simulink model "REPLAY_TRADITIONAL_21"  (R2021a)
settings: Solver=ode23tb  StartTime=0.0  StopTime=27  MaxStep=1/60  RelTol=1e-2  AbsTol=1e-1  EnableMultiTasking=on
PreLoadFcn:
  | NE39bus_data;
  | PSSMODEL=1;
  | LPSS=0;
  | WAPSS=0;
  | WAPSS2=0;
undefined symbols (not defined in the file): AVR_Data, D1, Delta, line, mac_con, MB, Ns, p0, Pn, s
libraries: spsThreePhaseVIMeasurementLib x40, spsThreePhasePISectionLineLib x34, spsGenericPowerSystemStabilizerLib x20, spsThreePhaseParallelRLCLoadLib x14, spsThreePhaseTransformerTwoWindingsLib x12, spsSynchronousMachinepuStandardLib x10, spsExcitationSystemLib x10, spsMultiBandPowerSystemStabilizerLib x10, spsSteamTurbineandGovernorLib x10, slpidlib x10, spsLoadFlowBusLib x9, spsThreePhaseBreakerLib x8
(part 2 of 4)

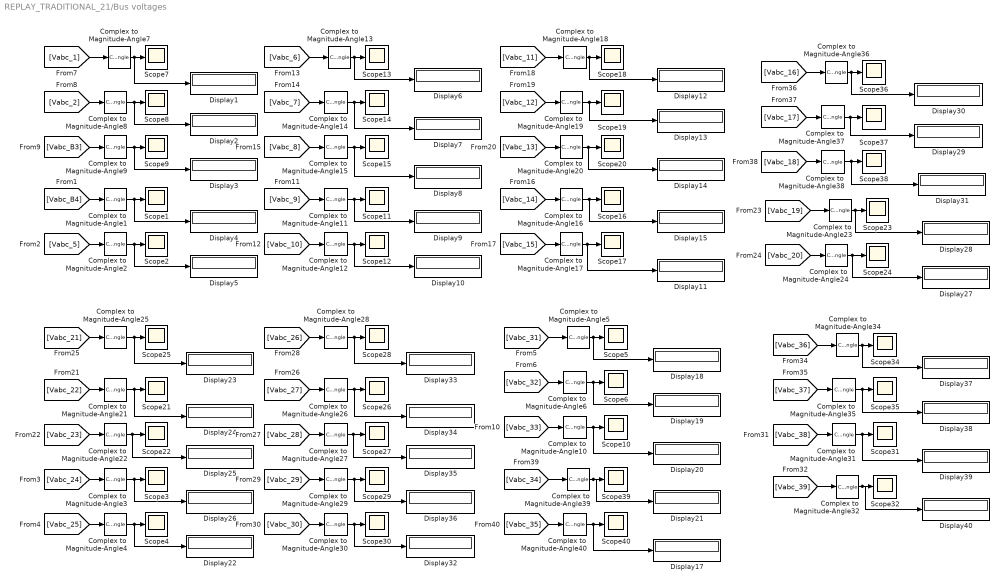
== system REPLAY_TRADITIONAL_21/Bus voltages ==
  Complex to Magnitude-Angle{1..32,34..40} (39 alike) : ComplexToMagnitudeAngle  Output=Magnitude
  Display{1..15,17..40} (39 alike) : Display
  Scope{1..32,34..40} (39 alike) : Scope
  wires:
  [Vabc_1] -> Complex to Magnitude-Angle7/1
  Complex to Magnitude-Angle7/1 -> Display1/1, Scope7/1
  [Vabc_2] -> Complex to Magnitude-Angle8/1
  Complex to Magnitude-Angle8/1 -> Display2/1, Scope8/1
  [Vabc_B3] -> Complex to Magnitude-Angle9/1
  Complex to Magnitude-Angle9/1 -> Display3/1, Scope9/1
  [Vabc_B4] -> Complex to Magnitude-Angle1/1
  Complex to Magnitude-Angle1/1 -> Display4/1, Scope1/1
  [Vabc_5] -> Complex to Magnitude-Angle2/1
  Complex to Magnitude-Angle2/1 -> Display5/1, Scope2/1
  [Vabc_31] -> Complex to Magnitude-Angle5/1
  [Vabc_32] -> Complex to Magnitude-Angle6/1
  [Vabc_33] -> Complex to Magnitude-Angle10/1
  [Vabc_24] -> Complex to Magnitude-Angle3/1
  [Vabc_25] -> Complex to Magnitude-Angle4/1
  [Vabc_6] -> Complex to Magnitude-Angle13/1
  [Vabc_7] -> Complex to Magnitude-Angle14/1
  [Vabc_8] -> Complex to Magnitude-Angle15/1
  [Vabc_9] -> Complex to Magnitude-Angle11/1
  [Vabc_10] -> Complex to Magnitude-Angle12/1
  [Vabc_11] -> Complex to Magnitude-Angle18/1
  Complex to Magnitude-Angle18/1 -> Display12/1, Scope18/1
  [Vabc_12] -> Complex to Magnitude-Angle19/1
  [Vabc_13] -> Complex to Magnitude-Angle20/1
  Complex to Magnitude-Angle20/1 -> Display14/1, Scope20/1
  [Vabc_14] -> Complex to Magnitude-Angle16/1
  Complex to Magnitude-Angle16/1 -> Display15/1, Scope16/1
  [Vabc_15] -> Complex to Magnitude-Angle17/1
  Complex to Magnitude-Angle17/1 -> Display11/1, Scope17/1
  [Vabc_19] -> Complex to Magnitude-Angle23/1
  [Vabc_20] -> Complex to Magnitude-Angle24/1
  [Vabc_21] -> Complex to Magnitude-Angle25/1
  [Vabc_22] -> Complex to Magnitude-Angle21/1
  [Vabc_23] -> Complex to Magnitude-Angle22/1
  Complex to Magnitude-Angle13/1 -> Display6/1, Scope13/1
  Complex to Magnitude-Angle14/1 -> Display7/1, Scope14/1
  Complex to Magnitude-Angle15/1 -> Display8/1, Scope15/1
  Complex to Magnitude-Angle11/1 -> Display9/1, Scope11/1
  Complex to Magnitude-Angle12/1 -> Display10/1, Scope12/1
  Complex to Magnitude-Angle19/1 -> Display13/1, Scope19/1
  [Vabc_16] -> Complex to Magnitude-Angle36/1
  [Vabc_17] -> Complex to Magnitude-Angle37/1
  [Vabc_18] -> Complex to Magnitude-Angle38/1
  Complex to Magnitude-Angle38/1 -> Display31/1, Scope38/1
  [Vabc_34] -> Complex to Magnitude-Angle39/1
  [Vabc_35] -> Complex to Magnitude-Angle40/1
  Complex to Magnitude-Angle5/1 -> Display18/1, Scope5/1
  Complex to Magnitude-Angle10/1 -> Display20/1, Scope10/1
  Complex to Magnitude-Angle39/1 -> Display21/1, Scope39/1
  Complex to Magnitude-Angle40/1 -> Display17/1, Scope40/1
  Complex to Magnitude-Angle6/1 -> Display19/1, Scope6/1
  Complex to Magnitude-Angle25/1 -> Display23/1, Scope25/1
  Complex to Magnitude-Angle22/1 -> Display25/1, Scope22/1
  Complex to Magnitude-Angle3/1 -> Display26/1, Scope3/1
  Complex to Magnitude-Angle4/1 -> Display22/1, Scope4/1
  Complex to Magnitude-Angle21/1 -> Display24/1, Scope21/1
  Complex to Magnitude-Angle23/1 -> Display28/1, Scope23/1
  Complex to Magnitude-Angle24/1 -> Display27/1, Scope24/1
  Complex to Magnitude-Angle36/1 -> Display30/1, Scope36/1
  Complex to Magnitude-Angle37/1 -> Display29/1, Scope37/1
  [Vabc_29] -> Complex to Magnitude-Angle29/1
  [Vabc_30] -> Complex to Magnitude-Angle30/1
  [Vabc_26] -> Complex to Magnitude-Angle28/1
  [Vabc_27] -> Complex to Magnitude-Angle26/1
  [Vabc_28] -> Complex to Magnitude-Angle27/1
  Complex to Magnitude-Angle28/1 -> Display33/1, Scope28/1
  Complex to Magnitude-Angle27/1 -> Display35/1, Scope27/1
  Complex to Magnitude-Angle29/1 -> Display36/1, Scope29/1
  Complex to Magnitude-Angle30/1 -> Display32/1, Scope30/1
  Complex to Magnitude-Angle26/1 -> Display34/1, Scope26/1
  [Vabc_36] -> Complex to Magnitude-Angle34/1
  [Vabc_37] -> Complex to Magnitude-Angle35/1
  [Vabc_38] -> Complex to Magnitude-Angle31/1
  [Vabc_39] -> Complex to Magnitude-Angle32/1
  Complex to Magnitude-Angle34/1 -> Display37/1, Scope34/1
  Complex to Magnitude-Angle31/1 -> Display39/1, Scope31/1
  Complex to Magnitude-Angle32/1 -> Display40/1, Scope32/1
  Complex to Magnitude-Angle35/1 -> Display38/1, Scope35/1

== system REPLAY_TRADITIONAL_21/G1 ==
  DFG1 : Inport
  Bus Selector : BusSelector  OutputSignals="Mechanical.Rotor speed deviation  dw (pu)"
  Bus to Vector : BusToVector
  Fcn2 : Fcn  Expr=60*(1+u)
  G1 : spsSynchronousMachinepuStandardLib/Synchronous Machine pu Standard  PresetModel=No  MechanicalLoad=Mechanical power Pm  ShowDetailedParameters=on  RotorType=Round  Units=per unit standard parameters  MeasurementBus=off  NominalParameters="[Pn(1,1)*1E9  345000   50 ]"  Reactances1="[mac_con(1,6:8)  mac_con(1,11:13)  mac_con(1,4)]"  Reactances2=[ 1.305, 0.296, 0.252, 0.474, 0.243, 0.18 ]  dAxisTimeConstants=Open-circuit  qAxisTimeConstants=Open-circuit  TimeConstants1=[]  TimeConstants2="[mac_con(1,9:10)  mac_con(1,14:15)]"  TimeConstants3=[]  TimeConstants4=[]  TimeConstants5=[ 1.01, 0.053, 0.1 ]  TimeConstants6=[]  TimeConstants7=[]  TimeConstants8=[]  StatorResistance=mac_con(1,5)  Mechanical="[ mac_con(1,16)  0  4]"  PolePairs=4  InitialConditions=[0 -53.3817 1.03438 1.03438 1.03438 11.5505 -108.45 131.55 1.07168]  SetSaturation=off  Saturation=[0.6404,0.7127,0.8441,0.9214,0.9956,1.082,1.19,1.316,1.457;0.7,0.7698,0.8872,0.9466,0.9969,1.046,1.1,1.151,1.201]  LoadFlowParameters=[1 1000000000 0 0 0]  TsPowergui=0  TsBlock=-1  IterativeModel=Forward Euler  IterativeDiscreteModel=Trapezoidal non iterative  BusType=PV  Pref=p0(1,1)*1E9  Qref=0  Qmin=-inf  Qmax=inf  PLF=0  QLF=0
      settings: SourceProductBaseCode=PS
  M1: Turbine & Regulators : Subsystem
  Matrix Multiply1 : Product  Multiplication=Matrix(*)
  Matrix Multiply2 : Product  Multiplication=Matrix(*)
  PID Controller : slpidlib/PID Controller  Controller=PID  Form=Parallel  TimeDomain=Continuous-time  UseExternalTs=off  SampleTime=-1  IntegratorMethod=Forward Euler  FilterMethod=Forward Euler  ControllerParametersSource=internal  P=-0.20298  I=1  D=0  UseFilter=on  N=100  TunerSelectOption=Frequency Response Based  InitialConditionSource=internal  InitialConditionForIntegrator=0  InitialConditionForFilter=0  DifferentiatorICPrevScaledInput=0  ExternalReset=none  TrackingMode=off  Kt=1  LimitOutput=off  SatLimitsSource=internal  UpperSaturationLimit=inf  LowerSaturationLimit=-inf  LinearizeAsGain=on  AntiWindupMode=none  Kb=1  POutMin=[]  POutMax=[]  IOutMin=[]  IOutMax=[]  DOutMin=[]  DOutMax=[]  NOutMin=[]  NOutMax=[]  SumOutMin=[]  SumOutMax=[]  SaturationOutMin=[]  SaturationOutMax=[]  PParamMin=[]  PParamMax=[]  IParamMin=[]  IParamMax=[]  DParamMin=[]  DParamMax=[]  NParamMin=[]  NParamMax=[]  KbParamMin=[]  KbParamMax=[]  KtParamMin=[]  KtParamMax=[]  KbOutMin=[]  KbOutMax=[]  KtOutMin=[]  KtOutMax=[]  IntegratorOutMin=[]  IntegratorOutMax=[]  FilterOutMin=[]  FilterOutMax=[]  SumI1OutMin=[]  SumI1OutMax=[]  SumI2OutMin=[]  SumI2OutMax=[]  SumI3OutMin=[]  SumI3OutMax=[]  SumI4OutMin=[]  SumI4OutMax=[]  SumDOutMin=[]  SumDOutMax=[]  DifferentiatorOutMin=[]  DifferentiatorOutMax=[]  FilterDiffOutCoefMin=[]  FilterDiffOutCoefMax=[]  ReciprocalOutMin=[]  ReciprocalOutMax=[]  SumDenOutMin=[]  SumDenOutMax=[]  SumNumOutMin=[]  SumNumOutMax=[]  DivideOutMin=[]  DivideOutMax=[]  UdiffTsProdOutMin=[]  UdiffTsProdOutMax=[]  NTsProdOutMin=[]  NTsProdOutMax=[]  UintegralTsProdOutMin=[]  UintegralTsProdOutMax=[]  UngainTsProdOutMin=[]  UngainTsProdOutMax=[]  IntegratorContinuousStateAttributes=''  IntegratorStateMustResolveToSignalObject=off  IntegratorRTWStateStorageClass=Auto  FilterContinuousStateAttributes=''  FilterStateMustResolveToSignalObject=off  FilterRTWStateStorageClass=Auto  ParallelPVariant=InternalParameters  IdealPVariant=Disabled  IVariant=InternalParameters  DVariant=InternalParameters  IntegratorVariant=Continuous  SatVariant=Disabled  AWVariant=Passthrough  PCopyVariant=Disabled  TRVariant=Disabled  FdbkBlocksVariant=Forward  IdealPFdbkVariant=Disabled  SatFdbkVariant=Disabled  DerivativeFilterVariant=ContFilter  NVariant=InternalParameters  NCopyVariant=Disabled  FilterICVariant=InternalICsFilter  IntegratorICVariant=InternalICs  ExternalResetVariant=Disabled  TRSumVariant=Passthrough  SumFdbkVariant=Disabled  SumVariant=Sum_PID  TsampFilterVariant=InternalTs  TsampNgainVariant=Passthrough  TsampIntegralVariant=Passthrough  ExternalSaturationOutDataTypeStr=Inherit: Same as second input
  Pref1 : Constant
  Scope3 : Scope
  Sum : Sum  Inputs=|++
  To Workspace : ToWorkspace  VariableName=average_frequency_39_bus  SaveFormat=Timeseries  SampleTime=-1
  Vref1 : Constant
  A : PMIOPort  Side=Left
  B : PMIOPort  Port=2  Side=Left
  C : PMIOPort  Port=3  Side=Left
  GEN1 : Outport
  wires:
  [PSSmodel] -> M1: Turbine & Regulators/4(PSS1)
  PID Controller/1 -> Sum/2
  Sum/1 -> M1: Turbine & Regulators/2(Pref1)
  Pref1/1 -> Sum/1
  Vref1/1 -> M1: Turbine & Regulators/3(Vref1)
  G1/1 -> Bus to Vector/1, M1: Turbine & Regulators/1(m), Bus Selector/1
  Bus Selector/1 -> Fcn2/1, PID Controller/1  "<Rotor speed deviation  dw (pu)>"
  Fcn2/1 -> GEN1/1, Scope3/1, To Workspace/1
  DFG1/1 -> Matrix Multiply1/1, Matrix Multiply2/1
  M1: Turbine & Regulators/1(Pm1) -> Matrix Multiply1/2
  Matrix Multiply1/1 -> G1/1
  M1: Turbine & Regulators/2(Vf1) -> Matrix Multiply2/2
  Matrix Multiply2/1 -> G1/2
  connections:
  A/RConn1 -- G1/RConn1
  B/RConn1 -- G1/RConn2
  C/RConn1 -- G1/RConn3

== system REPLAY_TRADITIONAL_21/G10 ==
  Inport : Inport
  Bus Selector : BusSelector  OutputSignals="Mechanical.Rotor speed deviation  dw (pu)"
  Fcn2 : Fcn  Expr=60*(1+u)
  G10 : spsSynchronousMachinepuStandardLib/Synchronous Machine pu Standard  PresetModel=No  MechanicalLoad=Mechanical power Pm  ShowDetailedParameters=on  RotorType=Round  Units=per unit standard parameters  MeasurementBus=off  NominalParameters="[Pn(10,1)*1E9  22000   50 ]"  Reactances1="[mac_con(10,6:8)  mac_con(10,11:13)  mac_con(10,4)]"  Reactances2=[ 1.305, 0.296, 0.252, 0.474, 0.243, 0.18 ]  dAxisTimeConstants=Open-circuit  qAxisTimeConstants=Open-circuit  TimeConstants1=[]  TimeConstants2="[mac_con(10,9:10)  mac_con(10,14:15)]"  TimeConstants3=[]  TimeConstants4=[]  TimeConstants5=[ 1.01, 0.053, 0.1 ]  TimeConstants6=[]  TimeConstants7=[]  TimeConstants8=[]  StatorResistance=mac_con(10,5)  Mechanical="[ mac_con(10,16)  0  4]"  PolePairs=4  InitialConditions=[0 -76.9944 0.265611 0.265611 0.265611 -15.9627 -135.963 104.037 1.1157]  SetSaturation=off  Saturation=[0.6404,0.7127,0.8441,0.9214,0.9956,1.082,1.19,1.316,1.457;0.7,0.7698,0.8872,0.9466,0.9969,1.046,1.1,1.151,1.201]  LoadFlowParameters=[1 250000000 0 0 0]  TsPowergui=0  TsBlock=-1  IterativeModel=Forward Euler  IterativeDiscreteModel=Trapezoidal non iterative  BusType=PV  Pref=p0(10,1)*1E9  Qref=0  Qmin=-inf  Qmax=inf  PLF=0  QLF=0
      settings: SourceProductBaseCode=PS
  M10: Turbine & Regulators : Subsystem
  Matrix Multiply1 : Product  Multiplication=Matrix(*)
  Matrix Multiply2 : Product  Multiplication=Matrix(*)
  PID Controller : slpidlib/PID Controller  Controller=PID  Form=Parallel  TimeDomain=Continuous-time  UseExternalTs=off  SampleTime=-1  IntegratorMethod=Forward Euler  FilterMethod=Forward Euler  ControllerParametersSource=internal  P=-0.20298  I=1  D=0  UseFilter=on  N=100  TunerSelectOption=Frequency Response Based  InitialConditionSource=internal  InitialConditionForIntegrator=0  InitialConditionForFilter=0  DifferentiatorICPrevScaledInput=0  ExternalReset=none  TrackingMode=off  Kt=1  LimitOutput=off  SatLimitsSource=internal  UpperSaturationLimit=inf  LowerSaturationLimit=-inf  LinearizeAsGain=on  AntiWindupMode=none  Kb=1  POutMin=[]  POutMax=[]  IOutMin=[]  IOutMax=[]  DOutMin=[]  DOutMax=[]  NOutMin=[]  NOutMax=[]  SumOutMin=[]  SumOutMax=[]  SaturationOutMin=[]  SaturationOutMax=[]  PParamMin=[]  PParamMax=[]  IParamMin=[]  IParamMax=[]  DParamMin=[]  DParamMax=[]  NParamMin=[]  NParamMax=[]  KbParamMin=[]  KbParamMax=[]  KtParamMin=[]  KtParamMax=[]  KbOutMin=[]  KbOutMax=[]  KtOutMin=[]  KtOutMax=[]  IntegratorOutMin=[]  IntegratorOutMax=[]  FilterOutMin=[]  FilterOutMax=[]  SumI1OutMin=[]  SumI1OutMax=[]  SumI2OutMin=[]  SumI2OutMax=[]  SumI3OutMin=[]  SumI3OutMax=[]  SumI4OutMin=[]  SumI4OutMax=[]  SumDOutMin=[]  SumDOutMax=[]  DifferentiatorOutMin=[]  DifferentiatorOutMax=[]  FilterDiffOutCoefMin=[]  FilterDiffOutCoefMax=[]  ReciprocalOutMin=[]  ReciprocalOutMax=[]  SumDenOutMin=[]  SumDenOutMax=[]  SumNumOutMin=[]  SumNumOutMax=[]  DivideOutMin=[]  DivideOutMax=[]  UdiffTsProdOutMin=[]  UdiffTsProdOutMax=[]  NTsProdOutMin=[]  NTsProdOutMax=[]  UintegralTsProdOutMin=[]  UintegralTsProdOutMax=[]  UngainTsProdOutMin=[]  UngainTsProdOutMax=[]  IntegratorContinuousStateAttributes=''  IntegratorStateMustResolveToSignalObject=off  IntegratorRTWStateStorageClass=Auto  FilterContinuousStateAttributes=''  FilterStateMustResolveToSignalObject=off  FilterRTWStateStorageClass=Auto  ParallelPVariant=InternalParameters  IdealPVariant=Disabled  IVariant=InternalParameters  DVariant=InternalParameters  IntegratorVariant=Continuous  SatVariant=Disabled  AWVariant=Passthrough  PCopyVariant=Disabled  TRVariant=Disabled  FdbkBlocksVariant=Forward  IdealPFdbkVariant=Disabled  SatFdbkVariant=Disabled  DerivativeFilterVariant=ContFilter  NVariant=InternalParameters  NCopyVariant=Disabled  FilterICVariant=InternalICsFilter  IntegratorICVariant=InternalICs  ExternalResetVariant=Disabled  TRSumVariant=Passthrough  SumFdbkVariant=Disabled  SumVariant=Sum_PID  TsampFilterVariant=InternalTs  TsampNgainVariant=Passthrough  TsampIntegralVariant=Passthrough  ExternalSaturationOutDataTypeStr=Inherit: Same as second input
  Pref10 : Constant  Value=0.25
  Scope : Scope
  Sum : Sum  Inputs=|+-
  Vref10 : Constant
  A : PMIOPort  Side=Left
  B : PMIOPort  Port=2  Side=Left
  C : PMIOPort  Port=3  Side=Left
  "GEN10 " : Outport
  wires:
  [PSSmodel] -> M10: Turbine & Regulators/4(PSS10)
  Vref10/1 -> M10: Turbine & Regulators/3(Vref10)
  G10/1 -> Bus Selector/1, M10: Turbine & Regulators/1(m)
  Bus Selector/1 -> PID Controller/1, Fcn2/1  "<Rotor speed deviation  dw (pu)>"
  Sum/1 -> M10: Turbine & Regulators/2(Pref10)
  Pref10/1 -> Sum/1
  PID Controller/1 -> Sum/2
  Fcn2/1 -> "GEN10 "/1, Scope/1
  Inport/1 -> Matrix Multiply2/1, Matrix Multiply1/1
  M10: Turbine & Regulators/1(Pm10) -> Matrix Multiply1/2
  Matrix Multiply1/1 -> G10/1
  M10: Turbine & Regulators/2(Vf10) -> Matrix Multiply2/2
  Matrix Multiply2/1 -> G10/2
  connections:
  A/RConn1 -- G10/RConn1
  B/RConn1 -- G10/RConn2
  C/RConn1 -- G10/RConn3

== system REPLAY_TRADITIONAL_21/G2 ==
  DFG2 : Inport
  Bus Selector : BusSelector  OutputSignals="Mechanical.Rotor speed deviation  dw (pu)"
  Fcn2 : Fcn  Expr=60*(1+u)
  G2 : spsSynchronousMachinepuStandardLib/Synchronous Machine pu Standard  PresetModel=No  MechanicalLoad=Mechanical power Pm  ShowDetailedParameters=on  RotorType=Round  Units=per unit standard parameters  MeasurementBus=off  NominalParameters="[Pn(2,1)*1E9  22000   50 ]"  Reactances1="[mac_con(2,6:8)  mac_con(2,11:13)  mac_con(2,4)]"  Reactances2=[ 1.305, 0.296, 0.252, 0.474, 0.243, 0.18 ]  dAxisTimeConstants=Open-circuit  qAxisTimeConstants=Open-circuit  TimeConstants1=[]  TimeConstants2="[mac_con(2,9:10)  mac_con(2,14:15)]"  TimeConstants3=[]  TimeConstants4=[]  TimeConstants5=[ 1.01, 0.053, 0.1 ]  TimeConstants6=[]  TimeConstants7=[]  TimeConstants8=[]  StatorResistance=mac_con(2,5)  Mechanical="[ mac_con(2,16)  0  4]"  PolePairs=4  InitialConditions=[0 -63.2657 0.339533 0.339533 0.339533 -35.2425 -155.242 84.7575 1.77729]  SetSaturation=off  Saturation=[0.6404,0.7127,0.8441,0.9214,0.9956,1.082,1.19,1.316,1.457;0.7,0.7698,0.8872,0.9466,0.9969,1.046,1.1,1.151,1.201]  LoadFlowParameters=[2 546000000 0 0 0]  TsPowergui=0  TsBlock=-1  IterativeModel=Forward Euler  IterativeDiscreteModel=Trapezoidal non iterative  BusType=swing  Pref=0  Qref=0  Qmin=-inf  Qmax=inf  PLF=0  QLF=0
      settings: SourceProductBaseCode=PS
  M2: Turbine & Regulators : Subsystem
  Matrix Multiply1 : Product  Multiplication=Matrix(*)
  Matrix Multiply2 : Product  Multiplication=Matrix(*)
  PID Controller : slpidlib/PID Controller  Controller=PID  Form=Parallel  TimeDomain=Continuous-time  UseExternalTs=off  SampleTime=-1  IntegratorMethod=Forward Euler  FilterMethod=Forward Euler  ControllerParametersSource=internal  P=-0.20298  I=1  D=0  UseFilter=on  N=100  TunerSelectOption=Frequency Response Based  InitialConditionSource=internal  InitialConditionForIntegrator=0  InitialConditionForFilter=0  DifferentiatorICPrevScaledInput=0  ExternalReset=none  TrackingMode=off  Kt=1  LimitOutput=off  SatLimitsSource=internal  UpperSaturationLimit=inf  LowerSaturationLimit=-inf  LinearizeAsGain=on  AntiWindupMode=none  Kb=1  POutMin=[]  POutMax=[]  IOutMin=[]  IOutMax=[]  DOutMin=[]  DOutMax=[]  NOutMin=[]  NOutMax=[]  SumOutMin=[]  SumOutMax=[]  SaturationOutMin=[]  SaturationOutMax=[]  PParamMin=[]  PParamMax=[]  IParamMin=[]  IParamMax=[]  DParamMin=[]  DParamMax=[]  NParamMin=[]  NParamMax=[]  KbParamMin=[]  KbParamMax=[]  KtParamMin=[]  KtParamMax=[]  KbOutMin=[]  KbOutMax=[]  KtOutMin=[]  KtOutMax=[]  IntegratorOutMin=[]  IntegratorOutMax=[]  FilterOutMin=[]  FilterOutMax=[]  SumI1OutMin=[]  SumI1OutMax=[]  SumI2OutMin=[]  SumI2OutMax=[]  SumI3OutMin=[]  SumI3OutMax=[]  SumI4OutMin=[]  SumI4OutMax=[]  SumDOutMin=[]  SumDOutMax=[]  DifferentiatorOutMin=[]  DifferentiatorOutMax=[]  FilterDiffOutCoefMin=[]  FilterDiffOutCoefMax=[]  ReciprocalOutMin=[]  ReciprocalOutMax=[]  SumDenOutMin=[]  SumDenOutMax=[]  SumNumOutMin=[]  SumNumOutMax=[]  DivideOutMin=[]  DivideOutMax=[]  UdiffTsProdOutMin=[]  UdiffTsProdOutMax=[]  NTsProdOutMin=[]  NTsProdOutMax=[]  UintegralTsProdOutMin=[]  UintegralTsProdOutMax=[]  UngainTsProdOutMin=[]  UngainTsProdOutMax=[]  IntegratorContinuousStateAttributes=''  IntegratorStateMustResolveToSignalObject=off  IntegratorRTWStateStorageClass=Auto  FilterContinuousStateAttributes=''  FilterStateMustResolveToSignalObject=off  FilterRTWStateStorageClass=Auto  ParallelPVariant=InternalParameters  IdealPVariant=Disabled  IVariant=InternalParameters  DVariant=InternalParameters  IntegratorVariant=Continuous  SatVariant=Disabled  AWVariant=Passthrough  PCopyVariant=Disabled  TRVariant=Disabled  FdbkBlocksVariant=Forward  IdealPFdbkVariant=Disabled  SatFdbkVariant=Disabled  DerivativeFilterVariant=ContFilter  NVariant=InternalParameters  NCopyVariant=Disabled  FilterICVariant=InternalICsFilter  IntegratorICVariant=InternalICs  ExternalResetVariant=Disabled  TRSumVariant=Passthrough  SumFdbkVariant=Disabled  SumVariant=Sum_PID  TsampFilterVariant=InternalTs  TsampNgainVariant=Passthrough  TsampIntegralVariant=Passthrough  ExternalSaturationOutDataTypeStr=Inherit: Same as second input
  Pref2 : Constant  Value=0.277303
  Scope : Scope
  Sum : Sum  Inputs=|+-
  Vref2 : Constant
  A : PMIOPort  Side=Left
  B : PMIOPort  Port=2  Side=Left
  C : PMIOPort  Port=3  Side=Left
  GEN2 : Outport
  wires:
  [PSSmodel] -> M2: Turbine & Regulators/4(PSS2)
  G2/1 -> Bus Selector/1, M2: Turbine & Regulators/1(m2)
  Bus Selector/1 -> PID Controller/1, Fcn2/1  "<Rotor speed deviation  dw (pu)>"
  PID Controller/1 -> Sum/2
  Vref2/1 -> M2: Turbine & Regulators/3(Vref2)
  Sum/1 -> M2: Turbine & Regulators/2(Pref2)
  Pref2/1 -> Sum/1
  Fcn2/1 -> GEN2/1, Scope/1
  DFG2/1 -> Matrix Multiply2/1, Matrix Multiply1/1
  M2: Turbine & Regulators/2(Vf2) -> Matrix Multiply2/2
  Matrix Multiply2/1 -> G2/2
  M2: Turbine & Regulators/1(Pm2) -> Matrix Multiply1/2
  Matrix Multiply1/1 -> G2/1
  connections:
  G2/RConn1 -- A/RConn1
  B/RConn1 -- G2/RConn2
  C/RConn1 -- G2/RConn3

== system REPLAY_TRADITIONAL_21/G3 ==
  DFG3 : Inport
  Bus Selector : BusSelector  OutputSignals="Mechanical.Rotor speed deviation  dw (pu)"
  Fcn2 : Fcn  Expr=60*(1+u)
  G3 : spsSynchronousMachinepuStandardLib/Synchronous Machine pu Standard  PresetModel=No  MechanicalLoad=Mechanical power Pm  ShowDetailedParameters=on  RotorType=Round  Units=per unit standard parameters  MeasurementBus=off  NominalParameters="[Pn(3,1)*1E9  22000   50 ]"  Reactances1="[mac_con(3,6:8)  mac_con(3,11:13)  mac_con(3,4)]"  Reactances2=[ 1.305, 0.296, 0.252, 0.474, 0.243, 0.18 ]  dAxisTimeConstants=Open-circuit  qAxisTimeConstants=Open-circuit  TimeConstants1=[]  TimeConstants2="[mac_con(3,9:10)  mac_con(3,14:15)]"  TimeConstants3=[]  TimeConstants4=[]  TimeConstants5=[ 1.01, 0.053, 0.1 ]  TimeConstants6=[]  TimeConstants7=[]  TimeConstants8=[]  StatorResistance=mac_con(3,5)  Mechanical="[ mac_con(3,16)  0  4]"  PolePairs=4  InitialConditions=[0 -37.958 0.689466 0.689466 0.689466 -12.356 -132.356 107.644 2.25944]  SetSaturation=off  Saturation=[0.6404,0.7127,0.8441,0.9214,0.9956,1.082,1.19,1.316,1.457;0.7,0.7698,0.8872,0.9466,0.9969,1.046,1.1,1.151,1.201]  LoadFlowParameters=[1 650000000 0 0 0]  TsPowergui=0  TsBlock=-1  IterativeModel=Forward Euler  IterativeDiscreteModel=Trapezoidal non iterative  BusType=PV  Pref=p0(3,1)*1E9  Qref=0  Qmin=-inf  Qmax=inf  PLF=0  QLF=0
      settings: SourceProductBaseCode=PS
  M3: Turbine & Regulators : Subsystem
  Matrix Multiply1 : Product  Multiplication=Matrix(*)
  Matrix Multiply2 : Product  Multiplication=Matrix(*)
  PID Controller : slpidlib/PID Controller  Controller=PID  Form=Parallel  TimeDomain=Continuous-time  UseExternalTs=off  SampleTime=-1  IntegratorMethod=Forward Euler  FilterMethod=Forward Euler  ControllerParametersSource=internal  P=-0.20298  I=1  D=0  UseFilter=on  N=100  TunerSelectOption=Frequency Response Based  InitialConditionSource=internal  InitialConditionForIntegrator=0  InitialConditionForFilter=0  DifferentiatorICPrevScaledInput=0  ExternalReset=none  TrackingMode=off  Kt=1  LimitOutput=off  SatLimitsSource=internal  UpperSaturationLimit=inf  LowerSaturationLimit=-inf  LinearizeAsGain=on  AntiWindupMode=none  Kb=1  POutMin=[]  POutMax=[]  IOutMin=[]  IOutMax=[]  DOutMin=[]  DOutMax=[]  NOutMin=[]  NOutMax=[]  SumOutMin=[]  SumOutMax=[]  SaturationOutMin=[]  SaturationOutMax=[]  PParamMin=[]  PParamMax=[]  IParamMin=[]  IParamMax=[]  DParamMin=[]  DParamMax=[]  NParamMin=[]  NParamMax=[]  KbParamMin=[]  KbParamMax=[]  KtParamMin=[]  KtParamMax=[]  KbOutMin=[]  KbOutMax=[]  KtOutMin=[]  KtOutMax=[]  IntegratorOutMin=[]  IntegratorOutMax=[]  FilterOutMin=[]  FilterOutMax=[]  SumI1OutMin=[]  SumI1OutMax=[]  SumI2OutMin=[]  SumI2OutMax=[]  SumI3OutMin=[]  SumI3OutMax=[]  SumI4OutMin=[]  SumI4OutMax=[]  SumDOutMin=[]  SumDOutMax=[]  DifferentiatorOutMin=[]  DifferentiatorOutMax=[]  FilterDiffOutCoefMin=[]  FilterDiffOutCoefMax=[]  ReciprocalOutMin=[]  ReciprocalOutMax=[]  SumDenOutMin=[]  SumDenOutMax=[]  SumNumOutMin=[]  SumNumOutMax=[]  DivideOutMin=[]  DivideOutMax=[]  UdiffTsProdOutMin=[]  UdiffTsProdOutMax=[]  NTsProdOutMin=[]  NTsProdOutMax=[]  UintegralTsProdOutMin=[]  UintegralTsProdOutMax=[]  UngainTsProdOutMin=[]  UngainTsProdOutMax=[]  IntegratorContinuousStateAttributes=''  IntegratorStateMustResolveToSignalObject=off  IntegratorRTWStateStorageClass=Auto  FilterContinuousStateAttributes=''  FilterStateMustResolveToSignalObject=off  FilterRTWStateStorageClass=Auto  ParallelPVariant=InternalParameters  IdealPVariant=Disabled  IVariant=InternalParameters  DVariant=InternalParameters  IntegratorVariant=Continuous  SatVariant=Disabled  AWVariant=Passthrough  PCopyVariant=Disabled  TRVariant=Disabled  FdbkBlocksVariant=Forward  IdealPFdbkVariant=Disabled  SatFdbkVariant=Disabled  DerivativeFilterVariant=ContFilter  NVariant=InternalParameters  NCopyVariant=Disabled  FilterICVariant=InternalICsFilter  IntegratorICVariant=InternalICs  ExternalResetVariant=Disabled  TRSumVariant=Passthrough  SumFdbkVariant=Disabled  SumVariant=Sum_PID  TsampFilterVariant=InternalTs  TsampNgainVariant=Passthrough  TsampIntegralVariant=Passthrough  ExternalSaturationOutDataTypeStr=Inherit: Same as second input
  Pref3 : Constant  Value=0.65
  Scope : Scope
  Sum : Sum  Inputs=|+-
  Vref3 : Constant
  A : PMIOPort  Side=Left
  B : PMIOPort  Port=2  Side=Left
  C : PMIOPort  Port=3  Side=Left
  GEN3 : Outport
  wires:
  G3/1 -> Bus Selector/1, M3: Turbine & Regulators/1(m3)
  Vref3/1 -> M3: Turbine & Regulators/3(Vref3)
  [PSSmodel] -> M3: Turbine & Regulators/4(PSS3)
  Bus Selector/1 -> PID Controller/1, Fcn2/1  "<Rotor speed deviation  dw (pu)>"
  Fcn2/1 -> GEN3/1, Scope/1
  Pref3/1 -> Sum/1
  Sum/1 -> M3: Turbine & Regulators/2(Pref3)
  PID Controller/1 -> Sum/2
  DFG3/1 -> Matrix Multiply2/1, Matrix Multiply1/1
  M3: Turbine & Regulators/1(Pm3) -> Matrix Multiply1/2
  Matrix Multiply1/1 -> G3/1
  M3: Turbine & Regulators/2(Vf3) -> Matrix Multiply2/2
  Matrix Multiply2/1 -> G3/2
  connections:
  A/RConn1 -- G3/RConn1
  B/RConn1 -- G3/RConn2
  C/RConn1 -- G3/RConn3

== system REPLAY_TRADITIONAL_21/G4 ==
  Bus Selector : BusSelector  OutputSignals="Mechanical.Rotor speed deviation  dw (pu)"
  Fcn2 : Fcn  Expr=60*(1+u)
  G4 : spsSynchronousMachinepuStandardLib/Synchronous Machine pu Standard  PresetModel=No  MechanicalLoad=Mechanical power Pm  ShowDetailedParameters=on  RotorType=Round  Units=per unit standard parameters  MeasurementBus=off  NominalParameters="[Pn(4,1)*1E9  22000   50 ]"  Reactances1="[mac_con(4,6:8)  mac_con(4,11:13)  mac_con(4,4)]"  Reactances2=[ 1.305, 0.296, 0.252, 0.474, 0.243, 0.18 ]  dAxisTimeConstants=Open-circuit  qAxisTimeConstants=Open-circuit  TimeConstants1=[]  TimeConstants2="[mac_con(4,9:10)  mac_con(4,14:15)]"  TimeConstants3=[]  TimeConstants4=[]  TimeConstants5=[ 1.01, 0.053, 0.1 ]  TimeConstants6=[]  TimeConstants7=[]  TimeConstants8=[]  StatorResistance=mac_con(4,5)  Mechanical="[ mac_con(4,16)  0  4]"  PolePairs=4  InitialConditions=[0 -27.7466 0.647548 0.647548 0.647548 -0.416201 -120.416 119.584 2.14879]  SetSaturation=off  Saturation=[0.6404,0.7127,0.8441,0.9214,0.9956,1.082,1.19,1.316,1.457;0.7,0.7698,0.8872,0.9466,0.9969,1.046,1.1,1.151,1.201]  LoadFlowParameters=[1 632000000 22000 0 0]  TsPowergui=0  TsBlock=-1  IterativeModel=Forward Euler  IterativeDiscreteModel=Trapezoidal non iterative  BusType=PV  Pref=p0(4,1)*1E9  Qref=0  Qmin=-inf  Qmax=inf  PLF=0  QLF=0
      settings: SourceProductBaseCode=PS
  M4: Turbine & Regulators : Subsystem
  PID Controller : slpidlib/PID Controller  Controller=PID  Form=Parallel  TimeDomain=Continuous-time  UseExternalTs=off  SampleTime=-1  IntegratorMethod=Forward Euler  FilterMethod=Forward Euler  ControllerParametersSource=internal  P=-0.20298  I=1  D=0  UseFilter=on  N=100  TunerSelectOption=Frequency Response Based  InitialConditionSource=internal  InitialConditionForIntegrator=0  InitialConditionForFilter=0  DifferentiatorICPrevScaledInput=0  ExternalReset=none  TrackingMode=off  Kt=1  LimitOutput=off  SatLimitsSource=internal  UpperSaturationLimit=inf  LowerSaturationLimit=-inf  LinearizeAsGain=on  AntiWindupMode=none  Kb=1  POutMin=[]  POutMax=[]  IOutMin=[]  IOutMax=[]  DOutMin=[]  DOutMax=[]  NOutMin=[]  NOutMax=[]  SumOutMin=[]  SumOutMax=[]  SaturationOutMin=[]  SaturationOutMax=[]  PParamMin=[]  PParamMax=[]  IParamMin=[]  IParamMax=[]  DParamMin=[]  DParamMax=[]  NParamMin=[]  NParamMax=[]  KbParamMin=[]  KbParamMax=[]  KtParamMin=[]  KtParamMax=[]  KbOutMin=[]  KbOutMax=[]  KtOutMin=[]  KtOutMax=[]  IntegratorOutMin=[]  IntegratorOutMax=[]  FilterOutMin=[]  FilterOutMax=[]  SumI1OutMin=[]  SumI1OutMax=[]  SumI2OutMin=[]  SumI2OutMax=[]  SumI3OutMin=[]  SumI3OutMax=[]  SumI4OutMin=[]  SumI4OutMax=[]  SumDOutMin=[]  SumDOutMax=[]  DifferentiatorOutMin=[]  DifferentiatorOutMax=[]  FilterDiffOutCoefMin=[]  FilterDiffOutCoefMax=[]  ReciprocalOutMin=[]  ReciprocalOutMax=[]  SumDenOutMin=[]  SumDenOutMax=[]  SumNumOutMin=[]  SumNumOutMax=[]  DivideOutMin=[]  DivideOutMax=[]  UdiffTsProdOutMin=[]  UdiffTsProdOutMax=[]  NTsProdOutMin=[]  NTsProdOutMax=[]  UintegralTsProdOutMin=[]  UintegralTsProdOutMax=[]  UngainTsProdOutMin=[]  UngainTsProdOutMax=[]  IntegratorContinuousStateAttributes=''  IntegratorStateMustResolveToSignalObject=off  IntegratorRTWStateStorageClass=Auto  FilterContinuousStateAttributes=''  FilterStateMustResolveToSignalObject=off  FilterRTWStateStorageClass=Auto  ParallelPVariant=InternalParameters  IdealPVariant=Disabled  IVariant=InternalParameters  DVariant=InternalParameters  IntegratorVariant=Continuous  SatVariant=Disabled  AWVariant=Passthrough  PCopyVariant=Disabled  TRVariant=Disabled  FdbkBlocksVariant=Forward  IdealPFdbkVariant=Disabled  SatFdbkVariant=Disabled  DerivativeFilterVariant=ContFilter  NVariant=InternalParameters  NCopyVariant=Disabled  FilterICVariant=InternalICsFilter  IntegratorICVariant=InternalICs  ExternalResetVariant=Disabled  TRSumVariant=Passthrough  SumFdbkVariant=Disabled  SumVariant=Sum_PID  TsampFilterVariant=InternalTs  TsampNgainVariant=Passthrough  TsampIntegralVariant=Passthrough  ExternalSaturationOutDataTypeStr=Inherit: Same as second input
  Pref4 : Constant  Value=0.632
  Scope : Scope
  Sum : Sum  Inputs=|++
  Vref4 : Constant
  A : PMIOPort  Side=Left
  B : PMIOPort  Port=2  Side=Left
  C : PMIOPort  Port=3  Side=Left
  GEN4 : Outport
  wires:
  G4/1 -> M4: Turbine & Regulators/1(m4), Bus Selector/1
  Vref4/1 -> M4: Turbine & Regulators/3(Vref4)
  [PSSmodel] -> M4: Turbine & Regulators/4(PSS4)
  M4: Turbine & Regulators/1(Pm4) -> G4/1
  M4: Turbine & Regulators/2(Vf4) -> G4/2
  Bus Selector/1 -> PID Controller/1, Fcn2/1  "<Rotor speed deviation  dw (pu)>"
  Fcn2/1 -> GEN4/1, Scope/1
  Pref4/1 -> Sum/1
  Sum/1 -> M4: Turbine & Regulators/2(Pref4)
  PID Controller/1 -> Sum/2
  connections:
  A/RConn1 -- G4/RConn1
  B/RConn1 -- G4/RConn2
  C/RConn1 -- G4/RConn3

== system REPLAY_TRADITIONAL_21/G5 ==
  Bus Selector : BusSelector  OutputSignals="Mechanical.Rotor speed deviation  dw (pu)"
  Compare To Constant : simulink/Logic and Bit Operations/Compare To Constant  relop=<=  const=58  OutDataTypeStr=boolean
  Compare To Constant1 : simulink/Logic and Bit Operations/Compare To Constant  relop=>=  const=62  OutDataTypeStr=boolean
  Fcn2 : Fcn  Expr=60*(1+u)
  G5 : spsSynchronousMachinepuStandardLib/Synchronous Machine pu Standard  PresetModel=No  MechanicalLoad=Mechanical power Pm  ShowDetailedParameters=on  RotorType=Round  Units=per unit standard parameters  MeasurementBus=off  NominalParameters="[Pn(5,1)*1E9  22000   50 ]"  Reactances1="[mac_con(5,6:8)  mac_con(5,11:13)  mac_con(5,4)]"  Reactances2=[ 1.305, 0.296, 0.252, 0.474, 0.243, 0.18 ]  dAxisTimeConstants=Open-circuit  qAxisTimeConstants=Open-circuit  TimeConstants1=[]  TimeConstants2="[mac_con(5,9:10)  mac_con(5,14:15)]"  TimeConstants3=[]  TimeConstants4=[]  TimeConstants5=[ 1.01, 0.053, 0.1 ]  TimeConstants6=[]  TimeConstants7=[]  TimeConstants8=[]  StatorResistance=mac_con(5,5)  Mechanical="[ mac_con(5,16)  0  4]"  PolePairs=4  InitialConditions=[0 -18.657 0.524928 0.524928 0.524928 -3.22796 -123.228 116.772 3.89055]  SetSaturation=off  Saturation=[0.6404,0.7127,0.8441,0.9214,0.9956,1.082,1.19,1.316,1.457;0.7,0.7698,0.8872,0.9466,0.9969,1.046,1.1,1.151,1.201]  LoadFlowParameters=[1 508000000 0 0 0]  TsPowergui=0  TsBlock=-1  IterativeModel=Forward Euler  IterativeDiscreteModel=Trapezoidal non iterative  BusType=PV  Pref=p0(5,1)*1E9  Qref=0  Qmin=-inf  Qmax=inf  PLF=0  QLF=0
      settings: SourceProductBaseCode=PS
  M5: Turbine & Regulators : Subsystem
  Matrix Multiply1 : Product  Multiplication=Matrix(*)
  Matrix Multiply2 : Product  Multiplication=Matrix(*)
  NOT : Logic  Operator=NOT  IconShape=distinctive  AllPortsSameDT=off  OutDataTypeStr=boolean
  OR : Logic  Operator=OR  IconShape=distinctive  AllPortsSameDT=off  OutDataTypeStr=boolean
  PID Controller : slpidlib/PID Controller  Controller=PID  Form=Parallel  TimeDomain=Continuous-time  UseExternalTs=off  SampleTime=-1  IntegratorMethod=Forward Euler  FilterMethod=Forward Euler  ControllerParametersSource=internal  P=-0.20298  I=1  D=0  UseFilter=on  N=100  TunerSelectOption=Frequency Response Based  InitialConditionSource=internal  InitialConditionForIntegrator=0  InitialConditionForFilter=0  DifferentiatorICPrevScaledInput=0  ExternalReset=none  TrackingMode=off  Kt=1  LimitOutput=off  SatLimitsSource=internal  UpperSaturationLimit=inf  LowerSaturationLimit=-inf  LinearizeAsGain=on  AntiWindupMode=none  Kb=1  POutMin=[]  POutMax=[]  IOutMin=[]  IOutMax=[]  DOutMin=[]  DOutMax=[]  NOutMin=[]  NOutMax=[]  SumOutMin=[]  SumOutMax=[]  SaturationOutMin=[]  SaturationOutMax=[]  PParamMin=[]  PParamMax=[]  IParamMin=[]  IParamMax=[]  DParamMin=[]  DParamMax=[]  NParamMin=[]  NParamMax=[]  KbParamMin=[]  KbParamMax=[]  KtParamMin=[]  KtParamMax=[]  KbOutMin=[]  KbOutMax=[]  KtOutMin=[]  KtOutMax=[]  IntegratorOutMin=[]  IntegratorOutMax=[]  FilterOutMin=[]  FilterOutMax=[]  SumI1OutMin=[]  SumI1OutMax=[]  SumI2OutMin=[]  SumI2OutMax=[]  SumI3OutMin=[]  SumI3OutMax=[]  SumI4OutMin=[]  SumI4OutMax=[]  SumDOutMin=[]  SumDOutMax=[]  DifferentiatorOutMin=[]  DifferentiatorOutMax=[]  FilterDiffOutCoefMin=[]  FilterDiffOutCoefMax=[]  ReciprocalOutMin=[]  ReciprocalOutMax=[]  SumDenOutMin=[]  SumDenOutMax=[]  SumNumOutMin=[]  SumNumOutMax=[]  DivideOutMin=[]  DivideOutMax=[]  UdiffTsProdOutMin=[]  UdiffTsProdOutMax=[]  NTsProdOutMin=[]  NTsProdOutMax=[]  UintegralTsProdOutMin=[]  UintegralTsProdOutMax=[]  UngainTsProdOutMin=[]  UngainTsProdOutMax=[]  IntegratorContinuousStateAttributes=''  IntegratorStateMustResolveToSignalObject=off  IntegratorRTWStateStorageClass=Auto  FilterContinuousStateAttributes=''  FilterStateMustResolveToSignalObject=off  FilterRTWStateStorageClass=Auto  ParallelPVariant=InternalParameters  IdealPVariant=Disabled  IVariant=InternalParameters  DVariant=InternalParameters  IntegratorVariant=Continuous  SatVariant=Disabled  AWVariant=Passthrough  PCopyVariant=Disabled  TRVariant=Disabled  FdbkBlocksVariant=Forward  IdealPFdbkVariant=Disabled  SatFdbkVariant=Disabled  DerivativeFilterVariant=ContFilter  NVariant=InternalParameters  NCopyVariant=Disabled  FilterICVariant=InternalICsFilter  IntegratorICVariant=InternalICs  ExternalResetVariant=Disabled  TRSumVariant=Passthrough  SumFdbkVariant=Disabled  SumVariant=Sum_PID  TsampFilterVariant=InternalTs  TsampNgainVariant=Passthrough  TsampIntegralVariant=Passthrough  ExternalSaturationOutDataTypeStr=Inherit: Same as second input
  Pref5 : Constant  Value=0.508
  Scope : Scope
  Sum : Sum  Inputs=|++
  Vref5 : Constant
  A : PMIOPort  Side=Left
  B : PMIOPort  Port=2  Side=Left
  C : PMIOPort  Port=3  Side=Left
  GEN5 : Outport
  wires:
  G5/1 -> Bus Selector/1, M5: Turbine & Regulators/1(m5)
  Vref5/1 -> M5: Turbine & Regulators/3(Vref5)
  [PSSmodel] -> M5: Turbine & Regulators/4(PSS5)
  Bus Selector/1 -> PID Controller/1, Fcn2/1  "<Rotor speed deviation  dw (pu)>"
  Fcn2/1 -> GEN5/1, Compare To Constant1/1, Compare To Constant/1, Scope/1
  Pref5/1 -> Sum/1
  PID Controller/1 -> Sum/2
  Sum/1 -> M5: Turbine & Regulators/2(Pref5)
  NOT/1 -> Matrix Multiply2/1, Matrix Multiply1/1
  M5: Turbine & Regulators/1(Pm5) -> Matrix Multiply1/2
  Matrix Multiply1/1 -> G5/1
  M5: Turbine & Regulators/2(Vf5) -> Matrix Multiply2/2
  Matrix Multiply2/1 -> G5/2
  Compare To Constant/1 -> OR/1
  Compare To Constant1/1 -> OR/2
  OR/1 -> NOT/1
  connections:
  G5/RConn1 -- A/RConn1
  G5/RConn2 -- B/RConn1
  G5/RConn3 -- C/RConn1

== system REPLAY_TRADITIONAL_21/G6 ==
  DFG6 : Inport
  Bus Selector : BusSelector  OutputSignals="Mechanical.Rotor speed deviation  dw (pu)"
  Fcn2 : Fcn  Expr=60*(1+u)
  G6 : spsSynchronousMachinepuStandardLib/Synchronous Machine pu Standard  PresetModel=No  MechanicalLoad=Mechanical power Pm  ShowDetailedParameters=on  RotorType=Round  Units=per unit standard parameters  MeasurementBus=off  NominalParameters="[Pn(6,1)*1E9  22000   50 ]"  Reactances1="[mac_con(6,6:8)  mac_con(6,11:13)  mac_con(6,4)]"  Reactances2=[ 1.305, 0.296, 0.252, 0.474, 0.243, 0.18 ]  dAxisTimeConstants=Open-circuit  qAxisTimeConstants=Open-circuit  TimeConstants1=[]  TimeConstants2="[mac_con(6,9:10)  mac_con(6,14:15)]"  TimeConstants3=[]  TimeConstants4=[]  TimeConstants5=[ 1.01, 0.053, 0.1 ]  TimeConstants6=[]  TimeConstants7=[]  TimeConstants8=[]  StatorResistance=mac_con(6,5)  Mechanical="[ mac_con(6,16)  0  4]"  PolePairs=4  InitialConditions=[0 -28.3893 0.677322 0.677322 0.677322 -1.75458 -121.755 118.245 2.21937]  SetSaturation=off  Saturation=[0.6404,0.7127,0.8441,0.9214,0.9956,1.082,1.19,1.316,1.457;0.7,0.7698,0.8872,0.9466,0.9969,1.046,1.1,1.151,1.201]  LoadFlowParameters=[1 650000000 0 0 0]  TsPowergui=0  TsBlock=-1  IterativeModel=Forward Euler  IterativeDiscreteModel=Trapezoidal non iterative  BusType=PV  Pref=p0(6,1)*1E9  Qref=0  Qmin=-inf  Qmax=inf  PLF=0  QLF=0
      settings: SourceProductBaseCode=PS
  M6: Turbine & Regulators : Subsystem
  Matrix Multiply1 : Product  Multiplication=Matrix(*)
  Matrix Multiply2 : Product  Multiplication=Matrix(*)
  NOT : Logic  Operator=NOT  IconShape=distinctive  AllPortsSameDT=off  OutDataTypeStr=boolean
  PID Controller : slpidlib/PID Controller  Controller=PID  Form=Parallel  TimeDomain=Continuous-time  UseExternalTs=off  SampleTime=-1  IntegratorMethod=Forward Euler  FilterMethod=Forward Euler  ControllerParametersSource=internal  P=-0.20298  I=1  D=0  UseFilter=on  N=100  TunerSelectOption=Frequency Response Based  InitialConditionSource=internal  InitialConditionForIntegrator=0  InitialConditionForFilter=0  DifferentiatorICPrevScaledInput=0  ExternalReset=none  TrackingMode=off  Kt=1  LimitOutput=off  SatLimitsSource=internal  UpperSaturationLimit=inf  LowerSaturationLimit=-inf  LinearizeAsGain=on  AntiWindupMode=none  Kb=1  POutMin=[]  POutMax=[]  IOutMin=[]  IOutMax=[]  DOutMin=[]  DOutMax=[]  NOutMin=[]  NOutMax=[]  SumOutMin=[]  SumOutMax=[]  SaturationOutMin=[]  SaturationOutMax=[]  PParamMin=[]  PParamMax=[]  IParamMin=[]  IParamMax=[]  DParamMin=[]  DParamMax=[]  NParamMin=[]  NParamMax=[]  KbParamMin=[]  KbParamMax=[]  KtParamMin=[]  KtParamMax=[]  KbOutMin=[]  KbOutMax=[]  KtOutMin=[]  KtOutMax=[]  IntegratorOutMin=[]  IntegratorOutMax=[]  FilterOutMin=[]  FilterOutMax=[]  SumI1OutMin=[]  SumI1OutMax=[]  SumI2OutMin=[]  SumI2OutMax=[]  SumI3OutMin=[]  SumI3OutMax=[]  SumI4OutMin=[]  SumI4OutMax=[]  SumDOutMin=[]  SumDOutMax=[]  DifferentiatorOutMin=[]  DifferentiatorOutMax=[]  FilterDiffOutCoefMin=[]  FilterDiffOutCoefMax=[]  ReciprocalOutMin=[]  ReciprocalOutMax=[]  SumDenOutMin=[]  SumDenOutMax=[]  SumNumOutMin=[]  SumNumOutMax=[]  DivideOutMin=[]  DivideOutMax=[]  UdiffTsProdOutMin=[]  UdiffTsProdOutMax=[]  NTsProdOutMin=[]  NTsProdOutMax=[]  UintegralTsProdOutMin=[]  UintegralTsProdOutMax=[]  UngainTsProdOutMin=[]  UngainTsProdOutMax=[]  IntegratorContinuousStateAttributes=''  IntegratorStateMustResolveToSignalObject=off  IntegratorRTWStateStorageClass=Auto  FilterContinuousStateAttributes=''  FilterStateMustResolveToSignalObject=off  FilterRTWStateStorageClass=Auto  ParallelPVariant=InternalParameters  IdealPVariant=Disabled  IVariant=InternalParameters  DVariant=InternalParameters  IntegratorVariant=Continuous  SatVariant=Disabled  AWVariant=Passthrough  PCopyVariant=Disabled  TRVariant=Disabled  FdbkBlocksVariant=Forward  IdealPFdbkVariant=Disabled  SatFdbkVariant=Disabled  DerivativeFilterVariant=ContFilter  NVariant=InternalParameters  NCopyVariant=Disabled  FilterICVariant=InternalICsFilter  IntegratorICVariant=InternalICs  ExternalResetVariant=Disabled  TRSumVariant=Passthrough  SumFdbkVariant=Disabled  SumVariant=Sum_PID  TsampFilterVariant=InternalTs  TsampNgainVariant=Passthrough  TsampIntegralVariant=Passthrough  ExternalSaturationOutDataTypeStr=Inherit: Same as second input
  Pref6 : Constant  Value=0.65
  Scope : Scope
  Sum : Sum  Inputs=|++
  Vref6 : Constant
  A : PMIOPort  Side=Left
  B : PMIOPort  Port=2  Side=Left
  C : PMIOPort  Port=3  Side=Left
  GEN6 : Outport
  wires:
  G6/1 -> Bus Selector/1, M6: Turbine & Regulators/1(m6)
  Vref6/1 -> M6: Turbine & Regulators/3(Vref6)
  [PSSmodel] -> M6: Turbine & Regulators/4(PSS6)
  Bus Selector/1 -> PID Controller/1, Fcn2/1  "<Rotor speed deviation  dw (pu)>"
  Fcn2/1 -> GEN6/1, Scope/1
  Pref6/1 -> Sum/1
  PID Controller/1 -> Sum/2
  Sum/1 -> M6: Turbine & Regulators/2(Pref6)
  DFG6/1 -> NOT/1
  NOT/1 -> Matrix Multiply2/1, Matrix Multiply1/1
  M6: Turbine & Regulators/1(Pm6) -> Matrix Multiply1/2
  Matrix Multiply1/1 -> G6/1
  M6: Turbine & Regulators/2(Vf6) -> Matrix Multiply2/2
  Matrix Multiply2/1 -> G6/2
  connections:
  A/RConn1 -- G6/RConn1
  B/RConn1 -- G6/RConn2
  C/RConn1 -- G6/RConn3

== system REPLAY_TRADITIONAL_21/G7 ==
  Bus Selector : BusSelector  OutputSignals="Mechanical.Rotor speed deviation  dw (pu)"
  Fcn2 : Fcn  Expr=60*(1+u)
  G7 : spsSynchronousMachinepuStandardLib/Synchronous Machine pu Standard  PresetModel=No  MechanicalLoad=Mechanical power Pm  ShowDetailedParameters=on  RotorType=Round  Units=per unit standard parameters  MeasurementBus=off  NominalParameters="[Pn(7,1)*1E9  22000   50 ]"  Reactances1="[mac_con(7,6:8)  mac_con(7,11:13)  mac_con(7,4)]"  Reactances2=[ 1.305, 0.296, 0.252, 0.474, 0.243, 0.18 ]  dAxisTimeConstants=Open-circuit  qAxisTimeConstants=Open-circuit  TimeConstants1=[]  TimeConstants2="[mac_con(7,9:10)  mac_con(7,14:15)]"  TimeConstants3=[]  TimeConstants4=[]  TimeConstants5=[ 1.01, 0.053, 0.1 ]  TimeConstants6=[]  TimeConstants7=[]  TimeConstants8=[]  StatorResistance=mac_con(7,5)  Mechanical="[ mac_con(7,16)  0  4]"  PolePairs=4  InitialConditions=[0 -22.3007 0.574969 0.574969 0.574969 4.77124 -115.229 124.771 2.15543]  SetSaturation=off  Saturation=[0.6404,0.7127,0.8441,0.9214,0.9956,1.082,1.19,1.316,1.457;0.7,0.7698,0.8872,0.9466,0.9969,1.046,1.1,1.151,1.201]  LoadFlowParameters=[1 560000000 0 0 0]  TsPowergui=0  TsBlock=-1  IterativeModel=Forward Euler  IterativeDiscreteModel=Trapezoidal non iterative  BusType=PV  Pref=p0(7,1)*1E9  Qref=0  Qmin=-inf  Qmax=inf  PLF=0  QLF=0
      settings: SourceProductBaseCode=PS
  M7: Turbine & Regulators : Subsystem
  PID Controller : slpidlib/PID Controller  Controller=PID  Form=Parallel  TimeDomain=Continuous-time  UseExternalTs=off  SampleTime=-1  IntegratorMethod=Forward Euler  FilterMethod=Forward Euler  ControllerParametersSource=internal  P=-0.20298  I=1  D=0  UseFilter=on  N=100  TunerSelectOption=Frequency Response Based  InitialConditionSource=internal  InitialConditionForIntegrator=0  InitialConditionForFilter=0  DifferentiatorICPrevScaledInput=0  ExternalReset=none  TrackingMode=off  Kt=1  LimitOutput=off  SatLimitsSource=internal  UpperSaturationLimit=inf  LowerSaturationLimit=-inf  LinearizeAsGain=on  AntiWindupMode=none  Kb=1  POutMin=[]  POutMax=[]  IOutMin=[]  IOutMax=[]  DOutMin=[]  DOutMax=[]  NOutMin=[]  NOutMax=[]  SumOutMin=[]  SumOutMax=[]  SaturationOutMin=[]  SaturationOutMax=[]  PParamMin=[]  PParamMax=[]  IParamMin=[]  IParamMax=[]  DParamMin=[]  DParamMax=[]  NParamMin=[]  NParamMax=[]  KbParamMin=[]  KbParamMax=[]  KtParamMin=[]  KtParamMax=[]  KbOutMin=[]  KbOutMax=[]  KtOutMin=[]  KtOutMax=[]  IntegratorOutMin=[]  IntegratorOutMax=[]  FilterOutMin=[]  FilterOutMax=[]  SumI1OutMin=[]  SumI1OutMax=[]  SumI2OutMin=[]  SumI2OutMax=[]  SumI3OutMin=[]  SumI3OutMax=[]  SumI4OutMin=[]  SumI4OutMax=[]  SumDOutMin=[]  SumDOutMax=[]  DifferentiatorOutMin=[]  DifferentiatorOutMax=[]  FilterDiffOutCoefMin=[]  FilterDiffOutCoefMax=[]  ReciprocalOutMin=[]  ReciprocalOutMax=[]  SumDenOutMin=[]  SumDenOutMax=[]  SumNumOutMin=[]  SumNumOutMax=[]  DivideOutMin=[]  DivideOutMax=[]  UdiffTsProdOutMin=[]  UdiffTsProdOutMax=[]  NTsProdOutMin=[]  NTsProdOutMax=[]  UintegralTsProdOutMin=[]  UintegralTsProdOutMax=[]  UngainTsProdOutMin=[]  UngainTsProdOutMax=[]  IntegratorContinuousStateAttributes=''  IntegratorStateMustResolveToSignalObject=off  IntegratorRTWStateStorageClass=Auto  FilterContinuousStateAttributes=''  FilterStateMustResolveToSignalObject=off  FilterRTWStateStorageClass=Auto  ParallelPVariant=InternalParameters  IdealPVariant=Disabled  IVariant=InternalParameters  DVariant=InternalParameters  IntegratorVariant=Continuous  SatVariant=Disabled  AWVariant=Passthrough  PCopyVariant=Disabled  TRVariant=Disabled  FdbkBlocksVariant=Forward  IdealPFdbkVariant=Disabled  SatFdbkVariant=Disabled  DerivativeFilterVariant=ContFilter  NVariant=InternalParameters  NCopyVariant=Disabled  FilterICVariant=InternalICsFilter  IntegratorICVariant=InternalICs  ExternalResetVariant=Disabled  TRSumVariant=Passthrough  SumFdbkVariant=Disabled  SumVariant=Sum_PID  TsampFilterVariant=InternalTs  TsampNgainVariant=Passthrough  TsampIntegralVariant=Passthrough  ExternalSaturationOutDataTypeStr=Inherit: Same as second input
  Pref7 : Constant  Value=0.56
  Scope : Scope
  Sum : Sum  Inputs=|+-
  Vref7 : Constant
  A : PMIOPort  Side=Left
  B : PMIOPort  Port=2  Side=Left
  C : PMIOPort  Port=3  Side=Left
  GEN7 : Outport
  wires:
  M7: Turbine & Regulators/1(Pm7) -> G7/1
  M7: Turbine & Regulators/2(Vf7) -> G7/2
  G7/1 -> Bus Selector/1, M7: Turbine & Regulators/1(m7)
  Vref7/1 -> M7: Turbine & Regulators/3(Vref7)
  [PSSmodel] -> M7: Turbine & Regulators/4(PSS7)
  Bus Selector/1 -> PID Controller/1, Fcn2/1  "<Rotor speed deviation  dw (pu)>"
  Fcn2/1 -> GEN7/1, Scope/1
  Pref7/1 -> Sum/1
  Sum/1 -> M7: Turbine & Regulators/2(Pref7)
  PID Controller/1 -> Sum/2
  connections:
  G7/RConn1 -- A/RConn1
  G7/RConn2 -- B/RConn1
  G7/RConn3 -- C/RConn1
